simulink model "Pouziti_Discontinuities"  (R2020b)
settings: Solver=VariableStepAuto  StartTime=0.0  StopTime=10.0  MaxStep=0.1  RelTol=1e-3  EnableMultiTasking=on
libraries: simulink x7
settings Model: Creator=Jirkovsk  LastModifiedBy=jirkovsky
settings DataIOCC: LimitDataPoints=on  SaveFormat=Array  ReturnWorkspaceOutputs=off
settings OptimizationCC: ExpressionDepthLimit=2147483647  LifeSpan=inf
settings DebuggingCC: ReadBeforeWriteMsg=DisableAll  WriteAfterWriteMsg=DisableAll  WriteAfterReadMsg=DisableAll  UnderspecifiedInitializationDetection=Classic  MergeDetectMultiDrivingBlocksExec=none  SolverPrmCheckMsg=warning  StateNameClashWarn=warning  SFUnexpectedBacktrackingDiag=warning  SFNoUnconditionalDefaultTransitionDiag=warning  SFExecutionAtInitializationDiag=none  ArithmeticOperatorsInVariantConditions=warning
settings HardwareCC: ProdBitPerPointer=32  ProdBitPerSizeT=32  ProdBitPerPtrDiffT=32  ProdLargestAtomicFloat=None  ProdIntDivRoundTo=Undefined  ProdEndianess=Unspecified  ProdWordSize=32  ProdHWDeviceType=32-bit Generic
settings ModelReferenceCC: PropagateSignalLabelsOutOfModel=off
settings SFSimCC: SimUseLocalCustomCode=off  CustomCodeUndefinedFunction=UseInterfaceOnly
settings RTWCC: RTWUseLocalCustomCode=off
settings CodeAppCC: StateflowObjectComments=on
settings GRTTargetCC: TargetLangStandard=C89/C90 (ANSI)
settings ConfigComp: CovMetricSettings=dw  CovSaveCumulativeToWorkspaceVar=on  CovSaveSingleToWorkspaceVar=on  CovExternalEMLEnable=off  CovSFcnEnable=off

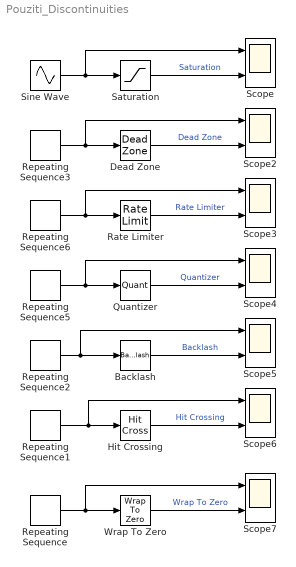
== system Pouziti_Discontinuities ==
  Backlash : Backlash  BacklashWidth=2
  Dead Zone : DeadZone  SaturateOnIntegerOverflow=on
  Hit Crossing : HitCross  HitCrossingOffset=5.35
  Quantizer : Quantizer  QuantizationInterval=1
  Rate Limiter : RateLimiter  SampleTimeMode=inherited
  Repeating Sequence : simulink/Sources/Repeating Sequence  rep_seq_t=[0 5 10]  rep_seq_y=[0 10 0]
  Repeating Sequence1 : simulink/Sources/Repeating Sequence  rep_seq_t=[0 5 10]  rep_seq_y=[0 10 0]
  Repeating Sequence2 : simulink/Sources/Repeating Sequence  rep_seq_t=[0 2 4 6 8 10]  rep_seq_y=[0 10 5 15 10 20]
  Repeating Sequence3 : simulink/Sources/Repeating Sequence  rep_seq_t=[0 5 10]  rep_seq_y=[-5 5 -5]
  Repeating Sequence5 : simulink/Sources/Repeating Sequence  rep_seq_t=[0 5 10]  rep_seq_y=[0 10 0]
  Repeating Sequence6 : simulink/Sources/Repeating Sequence  rep_seq_t=[0 3 6 8 10]  rep_seq_y=[0 3 0 3 0]
  Saturation : Saturate
  Scope{,2..7} (7 alike) : Scope  NumInputPorts=2
  Sine Wave : Sin  SampleTime=0
  Wrap To Zero : simulink/Discontinuities/Wrap To Zero  Threshold=5
      settings: SourceProductBaseCode=SL
  wires:
  Repeating Sequence/1 -> Scope7/1, Wrap To Zero/1
  Repeating Sequence1/1 -> Scope6/1, Hit Crossing/1
  Repeating Sequence2/1 -> Scope5/1, Backlash/1
  Hit Crossing/1 -> Scope6/2  "Hit Crossing"
  Backlash/1 -> Scope5/2  "Backlash"
  Wrap To Zero/1 -> Scope7/2  "Wrap To Zero"
  Sine Wave/1 -> Scope/1, Saturation/1
  Saturation/1 -> Scope/2  "Saturation"
  Repeating Sequence3/1 -> Scope2/1, Dead Zone/1
  Dead Zone/1 -> Scope2/2  "Dead Zone"
  Repeating Sequence5/1 -> Scope4/1, Quantizer/1
  Quantizer/1 -> Scope4/2  "Quantizer"
  Repeating Sequence6/1 -> Scope3/1, Rate Limiter/1
  Rate Limiter/1 -> Scope3/2  "Rate Limiter"
